simulink model "MotorPropellerModule"  (R2022a)
settings: Solver=VariableStepAuto  StartTime=0.0  StopTime=10.0  RelTol=1e-3
settings Model: DataDictionary=MiniDroneArchData.sldd  Creator=tshifera  LastModifiedBy=tshifera

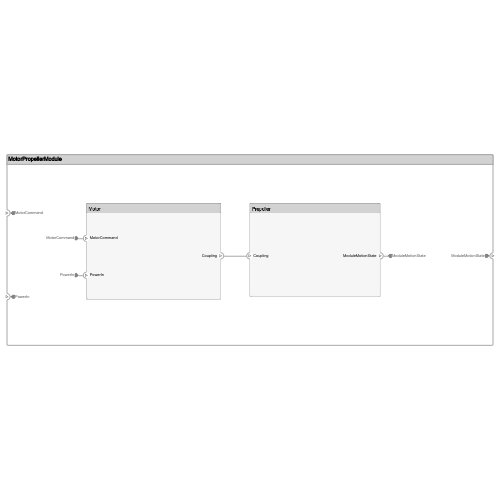
[thumbnail: Simulink's stored preview of the top-level diagram]
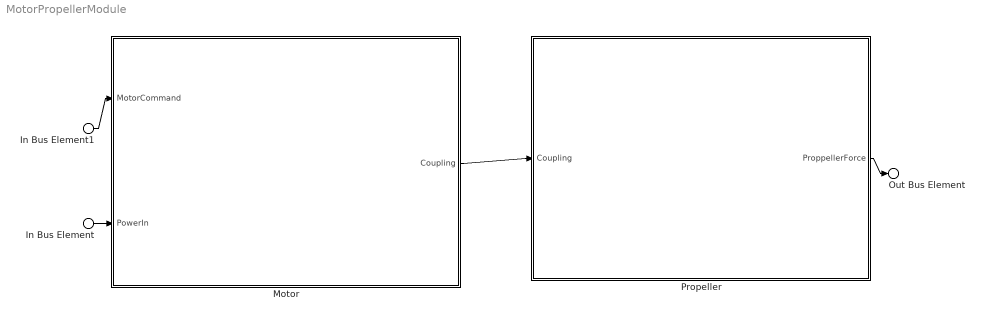
== system MotorPropellerModule ==
  In Bus Element1 : Inport  PortName=MotorCommand
  In Bus Element : Inport  Port=2  PortName=PowerIn
  Motor : Subsystem
      settings: PortSchema="{\"entries\":[{\"content\":{\"headerSize\":26,\"margin\":15,\"minimumSpacing\":25,\"sides\":[{\"content\":{\"connectorIds\":[\"In1\",\"In2\"]},\"type\":\"ConnectorPlacement.EquallySpacedRectSide\",\"uuid\":\"58971a95-43ec-4e42-90cb-f52848a43a78\"},{\"content\":{\"connectorIds\":[\"Out1\"],\"side\":\"RIGHT\"},\"type\":\"ConnectorPlacement.EquallySpacedRectSide\",\"uuid\":\"43bd139b-3ebd-443e-9d04-2758c166e5e5\"},{\"content\":{\"connectorIds\":[],\"side\":\"TOP\"},\"type\":\"ConnectorPlacement.EquallySpacedRectSide\",\"uuid\":\"9440dd5a-d47a-4e7e-9dec-7137884490cd\"}]},\"type\":\"ConnectorPlacement.EquallySpacedConnector\",\"uuid\":\"fbcd83c6-9a27-4688-9f1d-1a4d28d86620\"}],\"packageUris\":[\"http://schema.mathworks.com/mf0/Connector/R2020b\"],\"version\":\"1.0\"}"
  Propeller : Subsystem
      settings: PortSchema="{\"entries\":[{\"content\":{\"headerSize\":26,\"margin\":15,\"minimumSpacing\":25,\"sides\":[{\"content\":{\"connectorIds\":[\"In1\"]},\"type\":\"ConnectorPlacement.EquallySpacedRectSide\",\"uuid\":\"58971a95-43ec-4e42-90cb-f52848a43a78\"},{\"content\":{\"connectorIds\":[\"Out1\"],\"side\":\"RIGHT\"},\"type\":\"ConnectorPlacement.EquallySpacedRectSide\",\"uuid\":\"43bd139b-3ebd-443e-9d04-2758c166e5e5\"},{\"content\":{\"connectorIds\":[],\"side\":\"TOP\"},\"type\":\"ConnectorPlacement.EquallySpacedRectSide\",\"uuid\":\"9440dd5a-d47a-4e7e-9dec-7137884490cd\"}]},\"type\":\"ConnectorPlacement.EquallySpacedConnector\",\"uuid\":\"fbcd83c6-9a27-4688-9f1d-1a4d28d86620\"}],\"packageUris\":[\"http://schema.mathworks.com/mf0/Connector/R2020b\"],\"version\":\"1.0\"}"
  Out Bus Element : Outport  PortName=ProppellerForce
  wires:
  In Bus Element/1 -> Motor/2(PowerIn)
  Motor/1(Coupling) -> Propeller/1(Coupling)
  In Bus Element1/1 -> Motor/1(MotorCommand)
  Propeller/1(ProppellerForce) -> Out Bus Element/1

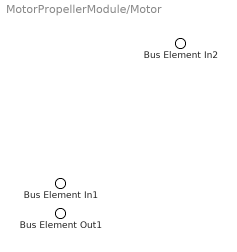
== system MotorPropellerModule/Motor ==
  Bus Element In2 : Inport  PortName=MotorCommand
  Bus Element In1 : Inport  Port=2  PortName=PowerIn
  Bus Element Out1 : Outport  PortName=Coupling

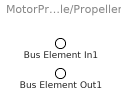
== system MotorPropellerModule/Propeller ==
  Bus Element In1 : Inport  PortName=Coupling
  Bus Element Out1 : Outport  PortName=ProppellerForce
